simulink model "steptest"  (R2014a)
settings: Solver=ode45  StartTime=0.0  StopTime=10.0  RelTol=1e-3
undefined symbols (not defined in the file): Humusoft, MF624
libraries: rtlib x3
settings Model: Creator=Administrador  LastModifiedBy=Administrador

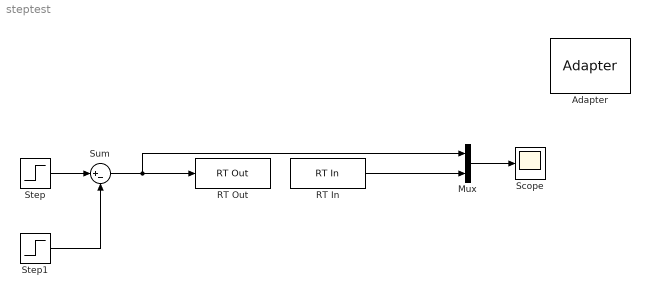
== system steptest ==
  Adapter : rtlib/Adapter  DriverName=Humusoft/MF624  DriverAddress=4294967295  DriverOptions=0
      settings: AttributesFormatString=Humusoft\nMF624 (auto)
  Mux : Mux  Inputs=2
  RT In : rtlib/RT In  SampleTime=0.01  Adapter=Adapter  IOClass=Analog Input  Channels=2  SLDataType=double  MaxMissedTicks=100  ShowMissedTicks=off  YieldWhenWaiting=on  AIORange=-10 to 10 V  AIOUnits=Volts  DIOMode=Bit  CIReset=never  CIEdge=rising  CIGate=none  EIQuadrature=quadruple  EIIndexPulse=reset  EIFilterFrequency=Inf  OIOParameters=[]
  RT Out : rtlib/RT Out  SampleTime=0.01  Adapter=Adapter  IOClass=Analog Output  Channels=2  InitialValue=[]  FinalValue=[]  MaxMissedTicks=100  ShowMissedTicks=off  YieldWhenWaiting=on  AIORange=-10 to 10 V  AIOUnits=Volts  DIOMode=Bit  OIOParameters=[]
  Scope : Scope
  Step : Step  After=5  SampleTime=0
  Step1 : Step  Time=8  After=5  SampleTime=0
  Sum : Sum  Inputs=|+-
  wires:
  Mux/1 -> Scope/1
  RT In/1 -> Mux/2
  Step/1 -> Sum/1
  Sum/1 -> Mux/1, RT Out/1
  Step1/1 -> Sum/2
